simulink model "P2001_230205_InstantaneousCostEM1_FromPaper"  (R2022b)
settings: Solver=VariableStepAuto  StartTime=0.0  StopTime=1  RelTol=1e-7
settings Model: Creator=turib  LastModifiedBy=turib

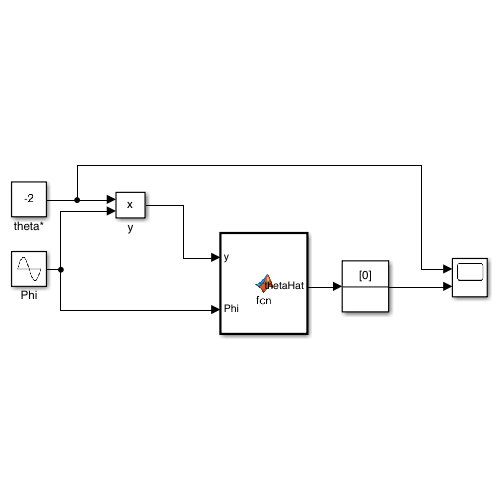
[thumbnail: Simulink's stored preview of the top-level diagram]
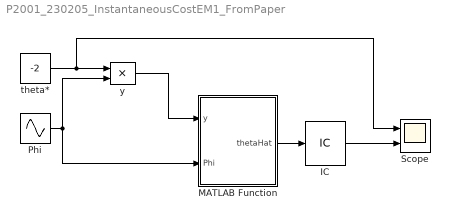
== system P2001_230205_InstantaneousCostEM1_FromPaper ==
  IC : InitialCondition  Value=0
  MATLAB Function : MATLAB Function  TreatAsAtomicUnit=on
  Phi : Sin  SampleTime=0
  Scope : Scope  NumInputPorts=2
  theta* : Constant  Value=-2
  y : Product  OutDataTypeStr=double
  wires:
  theta*/1 -> Scope/1, y/1
  Phi/1 -> MATLAB Function/2(Phi), y/2
  y/1 -> MATLAB Function/1(y)
  MATLAB Function/1(thetaHat) -> IC/1
  IC/1 -> Scope/2

== matlab function P2001_230205_InstantaneousCostEM1_FromPaper/MATLAB Function ==
  data: thetaHat output; y input; Phi input
function thetaHat  = fcn(y, Phi)
thetaHat = (Phi * Phi') ^ (-1) * (y * Phi');
end
